simulink model "Waypoint_Generator"  (R2017a)
settings: Solver=FixedStepAuto  StartTime=0.0  StopTime=50  FixedStep=0.005  RelTol=1e-3
libraries: dspbuff3 x1
settings Model: Creator=GusBus  LastModifiedBy=GusBus

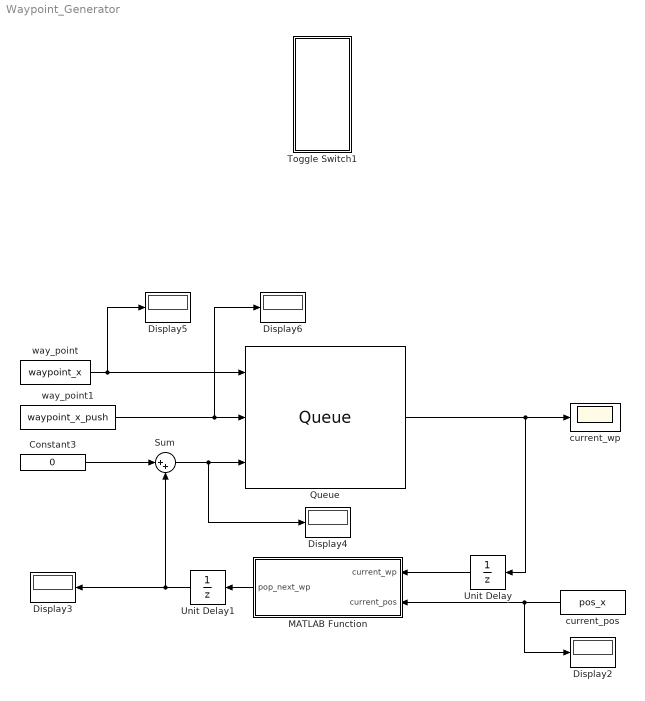
== system Waypoint_Generator ==
  Constant3 : Constant  Value=0
  Display{2..6} (5 alike) : Display
  MATLAB Function : MATLAB Function  TreatAsAtomicUnit=on
  Queue : dspbuff3/Queue  depth=64  trigger=Rising edge  overflow=Ignore  pes=Ignore  eso=off  fso=off  nso=off  clr=off  clrOutport=off  adf=on
      settings: SourceProductName=DSP System Toolbox  SourceProductBaseCode=DS
  Sum : Sum  Inputs=|++
  Toggle Switch1 : Subsystem  DialogController=hmiCreateDDGDialog  IsWebBlock=on  mask(MWDashboardBlock){webBlockId=e4ea970a-8c2f-4515-9ff2-5abf9519ff4b, webBlockType=toggleswitch, ShowInLibBrowser=on, ShowInitialText=on, HMISrcModelName=Waypoint_Generator}
      mask prompts: webBlockId "WebBlock Id"; webBlockType "WebBlock Type"; HMISrcModelName "Source Model"
      mask help: SimulinkHMI:dialogs:SwitchDialogDesc
      mask Help: helpview([docroot '/mapfiles/simulink.map'], 'hmi_toggle_switch')
      mask Display:
      | if strcmp(get_param(bdroot(gcb),'BlockDiagramType'), 'library')
      |     image([(matlabroot) '/toolbox/simulink/hmi/icons/ToggleSwitch.png']);
      | end
  Unit Delay : UnitDelay  SampleTime=-1
  Unit Delay1 : UnitDelay  SampleTime=0.1
  current_pos : FromWorkspace  VariableName=pos_x  SampleTime=0
  current_wp : Scope
  way_point : FromWorkspace  VariableName=waypoint_x  SampleTime=0  Interpolate=off  OutputAfterFinalValue=Holding final value
  way_point1 : FromWorkspace  VariableName=waypoint_x_push  SampleTime=0  Interpolate=off  OutputAfterFinalValue=Holding final value
  wires:
  way_point/1 -> Display5/1, Queue/1
  Queue/1 -> Unit Delay/1, current_wp/1
  MATLAB Function/1(pop_next_wp) -> Unit Delay1/1
  current_pos/1 -> Display2/1, MATLAB Function/2(current_pos)
  Unit Delay/1 -> MATLAB Function/1(current_wp)
  Sum/1 -> Display4/1, Queue/3
  Constant3/1 -> Sum/1
  Unit Delay1/1 -> Sum/2, Display3/1
  way_point1/1 -> Display6/1, Queue/2

== system Waypoint_Generator/Toggle Switch1 ==

== matlab function Waypoint_Generator/MATLAB Function ==
  data: current_wp input; current_pos input; pop_next_wp output
function pop_next_wp = fcn(current_wp, current_pos)

reached_waypoint_threshold = 0.25;                                             %metres, distance that confirms, wp has been reached

pop_next_wp = 0;

if abs(current_pos - current_wp) <= reached_waypoint_threshold              %If we have reached the threshold, trigger rising edge. I.e send out next waypoint
   pop_next_wp = 1;
end
